simulink model "sink"  (R2021b)
settings: Solver=FixedStepAuto  StartTime=0.0  StopTime=10.0  RelTol=1e-3
undefined symbols (not defined in the file or in its folder): f
libraries: instrumentlib x1
settings Model: DataDictionary=theSystem.sldd  Creator=samwarner  LastModifiedBy=samwarner

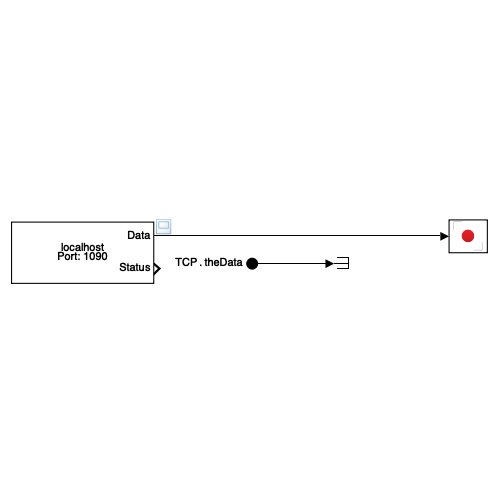
[thumbnail: Simulink's stored preview of the top-level diagram]
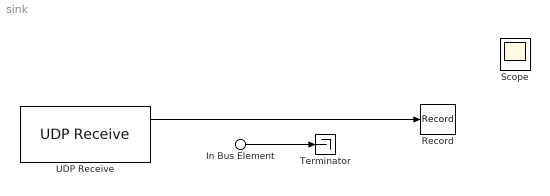
== system sink ==
  In Bus Element : Inport  PortName=TCP  Element=theData
  Record : Record  RecordToFile=on  FileSettingsInternal="{\"entries\":[{\"content\":{\"excelSettings\":{\"content\":{},\"type\":\"Streamout.ExcelSettings\"}},\"type\":\"Streamout.FileSettingStorage\",\"uuid\":\"ff6114f0-eb95-4b61-9719-e5e6e5de8a11\"}],\"packageUris\":[\"http://schema.mathworks.com/mf0/streamout_blocks/R2020a\"],\"version\":\"1.0\"}"  SignalsInternal="{\"entries\":[{\"content\":{\"signals\":[{\"content\":{\"blockPath\":[\"sink/Record\"],\"channel\":[],\"dimensions\":[1],\"domain\":\"sink/Record\",\"lineColor\":\"#edb120\",\"plots\":[1],\"port\":1,\"sid\":[],\"signalID\":9,\"signalName\":\"<theDaata>\"},\"type\":\"RecordBlkView.Signal\",\"uuid\":\"2a78b0e9-14cd-4996-8860-b38a5b86ba0a\"}]},\"type\":\"RecordBlkView.InputSignals\",\"uuid\":\"9318cc7f-0931-412b-b4a5-7070b9453faf\"},{\"content\":{\"signals\":[{\"content\":{\"blockPath\":[\"sink/Record\"],\"channel\":[],\"dimensions\":[1],\"domain\":\"sink/Record\",\"lineColor\":\"#edb120\",\"plots\":[],\"port\":1,\"sid\":[],\"signalID\":9,\"signalName\":\"<theDaata>\"},\"type\":\"RecordBlkView.Signal\",\"uuid\":\"01c9debf-5875-4655-b6c1-848bd30dfbb1\"}]},\"type\":\"RecordBlkView.InputSignals\",\"uuid\":\"acdf9e24-01d8-4bd2-b9a8-180e49c49441\"}],\"packageUris\":[\"http://schema.mathworks.com/mf0/streamout_blocks/R2020a\"],\"version\":\"1.0\"}"  VisualizationBindings="{\"sparklinesplugin\":{\"info\":[{\"bindingParametersList\":[],\"subplotID\":1}]}}"
  Terminator : Terminator
  UDP Receive : instrumentlib/UDP Receive  Host=localhost  Port=1091  LocalPort=1090  EnablePortSharing=on  GetLatestData=off  DataSize=[1 1]  DataType=uint8  ASCIIFormatting=%f,  Terminator=LF  ByteOrder=BigEndian  EnableBlockingMode=off  Timeout=10  SampleTime=-1  LocalAddress=localhost
  Scope : Scope
  wires:
  UDP Receive/1 -> Record/1
  In Bus Element/1 -> Terminator/1
